simulink model "LKAS_DFL_20210630"  (R2018b)
settings: Solver=FixedStepDiscrete  StartTime=0.0  StopTime=10.0  FixedStep=0.01  RelTol=1e-3
InitFcn:
  | tmpVer = ver('MATLAB');
  | tmpVer = str2num(tmpVer.Version);
  | % -------------------------------------------------------------------
  | %  MATLAB file generated by Simulink.saveVars on 21-Nov-2019 10:06:14
  | %  MATLAB version: 7.13.0.564 (R2011b)
  | % -------------------------------------------------------------------
  | 
  | 
  | SInt16 = Simulink.AliasType;
  | SInt16.Description = 'Num';
  | if (tmpVer > 7.11)
  | 	SInt16.DataScope = 'Auto';
  | end
  | SInt16.HeaderFile = 'Rte_Type.h';
  | SInt16.BaseType = 'int16';
  | 
  | SInt32 = Simulink.AliasType;
  | SInt32.Description = 'Num';
  | if (tmpVer > 7.11)
  | 	SInt32.DataScope = 'Auto';
  | end
  | SInt32.HeaderFile = 'Rte_Type.h';
  | SInt32.BaseType = 'int32';
  | 
  | SInt8 = Simulink.AliasType;
  | SInt8.Description = 'Num';
  | if (tmpVer > 7.11)
  | 	SInt8.DataScope = 'Auto';
  | end
  | SInt8.HeaderFile = 'Rte_Type.h';
  | SInt8.BaseType = 'int8';
  | 
  | T_A_m2_1024_1_u32 = Simulink.NumericType;
  | T_A_m2_1024_1_u32.Description = 'm2 (square meters  (m2))';
  | if (tmpVer > 7.11)
  | 	T_A_m2_1024_1_u32.DataScope = 'Auto';
  | end
  | T_A_m2_1024_1_u32.HeaderFile = 'Rte_Type.h';
  | T_A_m2_1024_1_u32.DataTypeMode = 'Fixed-point: slope and bias scaling';
  | T_A_m2_1024_1_u32.SignednessBool = false;
  | T_A_m2_1024_1_u32.WordLength = 32;
  | T_A_m2_1024_1_u32.FixedExponent = -10;
  | T_A_m2_1024_1_u32.SlopeAdjustmentFactor = 1;
  | T_A_m2_1024_1_u32.Bias = 0;
  | T_A_m2_1024_1_u32.DataTypeOverride = 'Inherit';
  | T_A_m2_1024_1_u32.IsAlias = true;
  | 
  | T_A_m2_65536_1_u16 = Simulink.NumericType;
  | T_A_m2_65536_1_u16.Description = 'm2 (square meters  (m2))';
  | if (tmpVer > 7.11)
  | 	T_A_m2_65536_1_u16.DataScope = 'Auto';
  | end
  | T_A_m2_65536_1_u16.HeaderFile = 'Rte_Type.h';
  | T_A_m2_65536_1_u16.DataTypeMode = 'Fixed-point: slope and bias scaling';
  | T_A_m2_65536_1_u16.SignednessBool = false;
  | T_A_m2_65536_1_u16.WordLength = 16;
  | T_A_m2_65536_1_u16.FixedExponent = -16;
  | T_A_m2_65536_1_u16.SlopeAdjustmentFactor = 1;
  | T_A_m2_65536_1_u16.Bias = 0;
  | T_A_m2_65536_1_u16.DataTypeOverride = 'Inherit';
  | ... (+4598 lines)
StopFcn:
  | clear  T_A_m2_1024_1_u32 T_A_m2_65536_1_u16 T_A_m2_Float32 T_A_mm2_10_1_u16 T_A_mm2_4_1_s16 T_A_mm2_Float32 T_Cnt_Num_10_1_u32 T_Cnt_Num_1_1_s16 T_Cnt_Num_1_1_s32 T_Cnt_Num_1_1_s8 T_Cnt_Num_1_1_u16 T_Cnt_Num_1_1_u32 T_Cnt_Num_1_1_u8 T_E_J_1_1_s32 T_E_J_Float32 T_E_kJ_128_1_s32 T_E_kJ_Float32 T_E_kwh_10_1_u16 T_E_kwh_Float32 T_Epl_kwhpkm_100_1_u16 T_Epl_kwhpkm_Float32 T_F_N_1_1_s16 T_F_N_Float32 T_I_A_1000_1_u16 T_I_A_1048576_1_s32 T_I_A_2048_1_s16 T_I_A_32_1_s16 T_I_A_Float32 T_I_mA_1_1_s16 T_I_mA_32768_128_s16 T_I_mA_Float32 T_J_kgpm2_128_1_u16 T_J_kgpm2_Float32 T_K_NA_1000_1_s16 T_K_NA_100_1_s16 T_K_NA_100_1_u16 T_K_NA_1024_1_s16 T_K_NA_1024_1_u16 T_K_NA_128_1_s16 T_K_NA_128_1_u16 T_K_NA_128_1_u8 T_K_NA_16777216_1_u32 T_K_NA_16_1_s16 T_K_NA_16_1_u16 T_K_NA_16_1_u8 T_K_NA_1_16_u16 T_K_NA_1_1_s16 T_K_NA_1_1_u16 T_K_NA_1_1_u8 T_K_NA_32768_1_s16 T_K_NA_32768_1_u16 T_K_NA_32_1_s8 T_K_NA_4096_1_u16 T_K_NA_4194304_1_s32 T_K_NA_4194304_1_u16 T_K_NA_65536_1_s32 T_K_NA_65536_1_u16 T_K_NA_8192_1_s16 T_K_NA_8_1_s16 T_K_NA_Float32 T_M_Nm_16_1_s16 T_M_Nm_1_1_s16 T_M_Nm_32768_1_s16 T_M_Nm_32_1_s16 T_M_Nm_4_1_s16 T_M_Nm_512_1_s16 T_M_Nm_Float32 T_P_W_1_4_s16 T_P_W_1_8_s16 T_P_W_Float32 T_P_kW_128_1_s16 T_P_kW_1_8_s16 T_P_kW_8_1_s32 T_P_kW_Float32 T_Pct_pct_1024_1_s32 T_Pct_pct_1024_1_u32 T_Pct_pct_10_1_s16 T_Pct_pct_10_1_u32 T_Pct_pct_128_100_s8 T_Pct_pct_1_1_s16 T_Pct_pct_1_4_u8 T_Pct_pct_255_100_u16 T_Pct_pct_255_100_u8 T_Pct_pct_256_1_s16 T_Pct_pct_256_1_u16 T_Pct_pct_65535_100_u16 T_Pct_pct_Float32 T_R_ohm_1024_1_s16 T_R_ohm_32_1_s16 T_R_ohm_Float32 T_TK_K_16_1_s16 T_TK_K_Float32 T_T_degC_10_400_1_u16 T_T_degC_16_1_s16 T_T_degC_1_40_1_u8 T_T_degC_2_80_1_u8 T_T_degC_Float32 T_U_V_1000_1_u16 T_U_V_10_1_u8 T_U_V_200_1_u8 T_U_V_32_1_s16 T_U_V_4096_1_s16 T_U_V_512_1_s16 T_U_V_65535_8_u16 T_U_V_8192_1_u16 T_U_V_Float32 T_U_mV_1_1_s16 T_U_mV_256_20_u16 T_U_mV_Float32 T_V_l_256_1_s16 T_V_l_4096_1_s16 T_V_l_64_1_s16 T_V_l_65535_100_u16 T_V_l_Float32 T_V_ml_128_1_s16 T_V_ml_1_1_s16 T_V_ml_32768_1_s16 T_V_ml_Float32 T_V_ul_32_1_u16 T_V_ul_Float32 T_Vpl_clpkm_512_1_u16 T_Vpl_clpkm_Float32 T_a_kphps_16_1_s16 T_a_kphps_Float32 T_a_mps2_128_1_s16 T_a_mps2_Float32 T_c_MJpkg_256_1_s16 T_c_MJpkg_Float32 T_c_kJpgpK_1024_1_s16 T_c_kJpgpK_Float32 T_c_kJpkgpK_128_1_u16 T_c_kJpkgpK_Float32 T_chrg_Ah_1_1_s16 T_chrg_Ah_1_1_u16 T_chrg_Ah_1_1_u8 T_chrg_Ah_256_1_u16 T_chrg_Ah_4194304_1_s32 T_chrg_Ah_512_1_u16 T_chrg_Ah_8_1_u16 T_chrg_Ah_Float32 T_cmp_NA_100_1_s16 T_cmp_NA_128_1_s16 T_cmp_NA_16_1_s16 T_cmp_NA_32768_1_u16 T_cmp_NA_Float32 T_d2n_rpmps2_4_1_s16 T_d2n_rpmps2_Float32 T_dPct_pctps_16_1_s16 T_dPct_pctps_256_1_s16 T_dPct_pctps_Float32 T_dT_degCps_128_1_s16 T_dT_degCps_Float32 T_dV_lph_1_1_s16 T_dV_lph_Float32 T_dV_lpm_128_1_s16 T_dV_lpm_32_1_s16 T_dV_lpm_Float32 T_dV_lps_1024_1_u16 T_dV_lps_4_1_u16 T_dV_lps_Float32 T_dV_mlps_1024_1_s16 T_dV_mlps_Float32 T_d_BitField16 T_dm_gps_128_1_s16 T_dm_gps_128_1_u16 T_dm_gps_256_1_u16 T_dm_gps_Float32 T_dm_mgps_1_1_s16 T_dm_mgps_Float32 T_dn_rpmps_1_1_s16 T_dn_rpmps_2_1_s16 T_dn_rpmps_Float32 T_dp_Paps_1_1_s16 T_dp_Paps_Float32 T_dp_kPaps_1_1_s16 T_dp_kPaps_8_1_s16 T_dp_kPaps_Float32 T_dphi_degps_128_1_s16 T_dphi_degps_8_1_s16 T_dphi_degps_Float32 T_dr_ps_256_1_s16 T_dr_ps_Float32 T_drho_mgplps_1_2_s16 T_drho_mgplps_Float32 T_e_NA_1_1_u8 T_f_Hz_1_1_u16 T_f_Hz_1_1_u32 T_f_Hz_64_1_u16 T_f_Hz_8_1_s16 T_f_Hz_Float32 T_g_BitField32 T_l_km_16_1_s16 T_l_km_1_1_u16 T_l_km_1_1_u32 T_l_km_Float32 T_l_m_1024_1_s16 T_l_m_16_1_s16 T_l_m_1_1_u32 T_l_m_Float32 T_l_mm_16_1_s16 T_l_mm_1_1_u16 T_l_mm_4096_1_s16 T_l_mm_4_1_u8 T_l_mm_64_1_s16 T_l_mm_Float32 T_m_g_1_1_s16 T_m_g_2048_1_s16 T_m_g_32_1_u16 T_m_g_Float32 T_m_kg_1024_1_s16 T_m_kg_1_1_s16 T_m_kg_1_1_u32 T_m_kg_Float32 T_m_mg_128_1_s16 T_m_mg_32_1_s16 T_m_mg_Float32 T_n_rpm_1_1_s16 T_n_rpm_1_25_u8 T_n_rpm_256_50_u16 T_n_rpm_2_25_u8 T_n_rpm_4_1_u16 T_n_rpm_Float32 T_p_MPa_64_1_s16 T_p_MPa_Float32 T_p_Pa_1_1_s16 T_p_Pa_Float32 T_p_kPa_1_10_u16 T_p_kPa_1_1_s16 T_p_kPa_1_1_u8 T_p_kPa_256_1_u16 T_p_kPa_32_1_u16 T_p_kPa_64_1_s16 T_p_kPa_Float32 T_phi_deg_100_1_s16 T_phi_deg_1024_1_s16 T_phi_deg_128_1_s16 T_phi_deg_1_1_u8 T_phi_deg_256_1_s16 T_phi_deg_2_1_s8 T_phi_deg_32_1_s16 T_phi_deg_512_6_s32 T_phi_deg_Float32 T_phi_rad_2048_1_s16 T_phi_rad_Float32 T_r_NA_1024_1_s16 T_r_NA_1024_1_u16 T_r_NA_16384_1_s16 T_r_NA_16_1_s16 T_r_NA_256_1_s8 T_r_NA_256_1_u16 T_r_NA_32768_1_u16 T_r_NA_32_1_u16 T_r_NA_4096_1_s16 T_r_NA_65535_2_u16 T_r_NA_8192_1_u16 T_r_NA_Float32 T_rho_gpl_8192_1_s16 T_rho_gpl_Float32 T_rho_kgpm3_16_1_s16 T_rho_kgpm3_Float32 T_rho_mgpl_1_1_s16 T_rho_mgpl_64_1_s16 T_rho_mgpl_Float32 T_t_hour_1_1_s16 T_t_hour_Float32 T_t_m_1_1_u16 T_t_m_Float32 T_t_ms_1_1_s16 T_t_ms_1_1_u16 T_t_ms_1_1_u32 T_t_ms_4096_1_s16 T_t_ms_64_1_s16 T_t_ms_Float32 T_t_s_1000_1_s16 T_t_s_100_1_s16 T_t_s_10_1_s16 T_t_s_10_1_u16 T_t_s_1_1_s16 T_t_s_1_1_u16 T_t_s_1_1_u32 T_t_s_Float32 T_t_us_10_1_u32 T_t_us_1_1_s16 T_t_us_1_1_u32 T_t_us_1_4_u16 T_t_us_Float32 T_v_kph_1_1_u8 T_v_kph_64_1_s16 T_v_kph_64_1_u16 T_v_kph_Float32 T_v_mps_256_1_s16 T_v_mps_Float32 T_w_radps_32_1_s16 T_w_radps_Float32 T_y_BitField8 T_y_BitFieldDiagProgress T_y_BitFieldDiagStatus T_y_NA_1_1_u8 SInt16 SInt32 SInt8 T_BOOLEAN UInt16 UInt32 UInt8 s16 s32 s8 u16 u32 u8
model workspace (MAT data in the model file):
  MCOS : class17 (value not decoded)
  MCOS : class17 (value not decoded)
  MCOS : class17 (value not decoded)
  MCOS : class17 (value not decoded)
  MCOS : class17 (value not decoded)
  MCOS : class17 (value not decoded)
  MCOS : class17 (value not decoded)
  MCOS : class17 (value not decoded)
  MCOS : class17 (value not decoded)
  MCOS : class17 (value not decoded)
  MCOS : class17 (value not decoded)
  MCOS : class17 (value not decoded)
  MCOS : class17 (value not decoded)
  MCOS : class17 (value not decoded)
  MCOS : class17 (value not decoded)
  MCOS : class17 (value not decoded)
  MCOS : class17 (value not decoded)
  MCOS : class17 (value not decoded)
  MCOS : class17 (value not decoded)
  MCOS : class17 (value not decoded)
  MCOS : class17 (value not decoded)
  MCOS : class17 (value not decoded)
  MCOS : class17 (value not decoded)
  MCOS : class17 (value not decoded)
  MCOS : class17 (value not decoded)
  MCOS : class17 (value not decoded)
  MCOS : class17 (value not decoded)
  MCOS : class17 (value not decoded)
  MCOS : class17 (value not decoded)
  MCOS : class17 (value not decoded)
  MCOS : class17 (value not decoded)
  MCOS : class17 (value not decoded)
  MCOS : class17 (value not decoded)
  MCOS : class17 (value not decoded)
  MCOS : class17 (value not decoded)
  MCOS : class17 (value not decoded)
  MCOS : class17 (value not decoded)
  MCOS : class17 (value not decoded)
  MCOS : class17 (value not decoded)
  MCOS : class17 (value not decoded)
  MCOS : class17 (value not decoded)
  MCOS : class17 (value not decoded)
  MCOS : class17 (value not decoded)
  MCOS : class17 (value not decoded)
  MCOS : class17 (value not decoded)
  MCOS : class17 (value not decoded)
  MCOS : class17 (value not decoded)
  MCOS : class17 (value not decoded)
  MCOS : class17 (value not decoded)
  MCOS : class17 (value not decoded)
  MCOS : class17 (value not decoded)
  MCOS : class17 (value not decoded)
  MCOS : class17 (value not decoded)
  MCOS : class17 (value not decoded)
  MCOS : class17 (value not decoded)
  MCOS : class17 (value not decoded)
  MCOS : class17 (value not decoded)
  MCOS : class17 (value not decoded)
  MCOS : class17 (value not decoded)
  MCOS : class17 (value not decoded)
  MCOS : class17 (value not decoded)
  MCOS : class17 (value not decoded)
  MCOS : class17 (value not decoded)
  MCOS : class17 (value not decoded)
  MCOS : class17 (value not decoded)
  MCOS : class17 (value not decoded)
  MCOS : class17 (value not decoded)
  MCOS : class17 (value not decoded)
  MCOS : class17 (value not decoded)
  MCOS : class17 (value not decoded)
  MCOS : class17 (value not decoded)
  MCOS : class17 (value not decoded)
  MCOS : class17 (value not decoded)
  MCOS : class17 (value not decoded)
  MCOS : class17 (value not decoded)
  MCOS : class17 (value not decoded)
  MCOS : class17 (value not decoded)
  MCOS : class17 (value not decoded)
  MCOS : class17 (value not decoded)
  MCOS : class17 (value not decoded)
  MCOS : class17 (value not decoded)
  MCOS : class17 (value not decoded)
  MCOS : class17 (value not decoded)
  MCOS : class17 (value not decoded)
  MCOS : class17 (value not decoded)
  MCOS : class17 (value not decoded)
  MCOS : class17 (value not decoded)
  MCOS : class17 (value not decoded)
  MCOS : class17 (value not decoded)
  MCOS : class17 (value not decoded)
  MCOS : class17 (value not decoded)
  MCOS : class17 (value not decoded)
  MCOS : class17 (value not decoded)
  MCOS : class17 (value not decoded)
  MCOS : class17 (value not decoded)
undefined symbols (not defined in the file): LKA_CarWidth, LKA_SampleTime, LKA_StrRatio_C, LKA_Veh2CamL_C, LKA_Veh2CamW_C, LKA_WhlBaseL_C, LL_CompSWA_C, LL_CrvtPrvwT_C, LL_DesDvt_C, LL_DvtComp_C, LL_DvtPrvwT_C, LL_DvtSpdDet_vDvtSpdMin_C, LL_HdAgExT_C, LL_HdAgPrvwT_C, LL_LAccMax_C, LL_LAccRMax_C, LL_Laneline_Select, LL_LDW_EarliestWarnLine_C, LL_LDW_LatestWarnLine_C, LL_LDWS_SUPPRESS_HEADING, LL_LFClb_TFC_DiffCtlBalance, LL_LFClb_TFC_DiffCtrlMaxSWA, LL_LFClb_TFC_DiffCtrlRatio, LL_LFClb_TFC_facmGainLutGain1_C, LL_LFClb_TFC_facmGainLutGain2_C, LL_LFClb_TFC_facmIntegRatio, LL_LFClb_TFC_facmKlat_C, LL_LFClb_TFC_FfCtlRatio_C, LL_LFClb_TFC_phiIntegCtlMaxSWA_C, LL_LFClb_TFC_tiKlatPrvwT_C, LL_LFClb_TFC_vGainLutVehSpdLwr_C, LL_LFClb_TFC_vGainLutVehSpdUpr_C, LL_LKA_EarliestWarnLine_C, LL_LKA_LatestWarnLine_C, LL_LKAExPrcs_ExitC0Dvt, LL_LKAExPrcs_ExitC0Swt, LL_LKAExPrcs_tiExitTime1, LL_LKAExPrcs_tiExitTime2, LL_LKAExPrcs_tiExitTime3, LL_LKAS_OUT_OF_CONTROL_LAT_VEL, LL_LKAS_OUT_OF_CONTROL_TTLC, LL_LKASWASyn_M0, LL_LKASWASyn_M1, LL_LKASWASyn_M2, LL_LKASWASyn_M3K, LL_LKASWASyn_SWAaddMax, LL_LKASWASyn_T2, LL_LKASWASyn_tiTrqSwaRtTime, LL_LKASWASyn_tiTrqSwaTime, LL_LKASWASyn_TrqMax, LL_LKASWASyn_TrqSwaAddSwt, LL_LKASWASyn_TrqSwaRateDiff, LL_LSpdCompT_C, LL_lStpLngth_C, LL_MAX_DELAY_EPSSTAR_TIME, LL_MAX_DRIVER_TORQUE_DISABLE, LL_MAX_DRIVER_TORQUE_ENABLE, LL_MAX_LANE_WIDTH_DISABLE, LL_MAX_LANE_WIDTH_ENABLE, LL_MAX_LAT_ACC_DISABLE ... (+35)
libraries: simulink x130, dspstat3 x3, simulink_extras x1
(part 6 of 18)

== system LKAS_DFL_20210630/LKAS/LL/LL Inputs Mapping/bsBCMInfo ==
  note: <BCM_Double_Light>
      | 0:off
      | 1:on
  note: <BCM_Left_Light>
      | 0:off
      | 1:on
  note: <BCM_Right_Light>
      | 0:off
      | 1:on
  bsBCMInfoIn : Inport
  Bus Creator1 : BusCreator  Inputs=3
  Bus Selector1 : BusSelector  OutputSignals=BCM_Double_Light,BCM_Left_Light,BCM_Right_Light
  bsBCMInfoOut : Outport
  wires:
  Bus Selector1/3 -> Bus Creator1/3  "<BCM_Right_Light>"
  Bus Selector1/2 -> Bus Creator1/2  "<BCM_Left_Light>"
  Bus Creator1/1 -> bsBCMInfoOut/1
  Bus Selector1/1 -> Bus Creator1/1  "<BCM_Double_Light>"
  bsBCMInfoIn/1 -> Bus Selector1/1

== system LKAS_DFL_20210630/LKAS/LL/LL Inputs Mapping/bsEPSInfo ==
  note: <EPS_LKA_State>
      | 0:init
      | 1:authorized
      | 2:wait
      | 3:active
      | 4:fault
  note: <EPS_Error_State>
      | 0:no error
      | 1:error
  note: <EPS_Trq_State>
      | 0:no error
      | 1:error
  note: <SAS_Clb_State>
      | 0:no clb
      | 1:clb
  note: <SAS_Trim_State>
      | 0:no trim
      | 1:trim
  note: <EPS_TrqLim_State>
      | 0:no limit
      | 1:limit
  note: <EPS_SWHold_State>
      | 0:no hold
      | 1:hold
  bsEPSInfoIn : Inport
  Bus Creator4 : BusCreator  Inputs=9
  Bus Selector1 : BusSelector  OutputSignals=EPS_LKA_State,EPS_SW_Trq,EPS_Error_State,EPS_Trq_State,SAS_Clb_State,SAS_Trim_State,EPS_TrqLim_State,EPS_LKA_Current,EPS_SWHold_State
  bsEPSInfoOut : Outport
  wires:
  Bus Selector1/9 -> Bus Creator4/9  "<EPS_SWHold_State>"
  Bus Selector1/8 -> Bus Creator4/8  "<EPS_LKA_Current>"
  Bus Selector1/7 -> Bus Creator4/7  "<EPS_TrqLim_State>"
  Bus Selector1/6 -> Bus Creator4/6  "<SAS_Trim_State>"
  Bus Selector1/5 -> Bus Creator4/5  "<SAS_Clb_State>"
  Bus Selector1/4 -> Bus Creator4/4  "<EPS_Trq_State>"
  Bus Selector1/3 -> Bus Creator4/3  "<EPS_Error_State>"
  Bus Creator4/1 -> bsEPSInfoOut/1
  Bus Selector1/1 -> Bus Creator4/1  "<EPS_LKA_State>"
  Bus Selector1/2 -> Bus Creator4/2  "<EPS_SW_Trq>"
  bsEPSInfoIn/1 -> Bus Selector1/1

== system LKAS_DFL_20210630/LKAS/LL/LL Inputs Mapping/bsLaneInfo ==
  bsLaneInfoIn : Inport
  Bus Creator : BusCreator  Inputs=7
  Bus Selector1 : BusSelector  OutputSignals=bsFusLaneInfo,bsFusL0Info,bsFusR0Info,bsFusL1Info,bsFusR1Info,bsOriLaneInfo,bsOriL0Info,bsOriR0Info,bsOriL1Info,bsOriR1Info,Fusion_AdditionalInf
  LaneSelect : Subsystem
  "LanesReconstruct " : Subsystem
  bsLaneInfoOut : Outport
  wires:
  Bus Selector1/1 -> Bus Creator/1  "<bsFusLaneInfo>"
  Bus Selector1/6 -> Bus Creator/6  "<bsOriLaneInfo>"
  Bus Creator/1 -> bsLaneInfoOut/1
  Bus Selector1/10 -> LaneSelect/8(bsOriR1Info)  "<bsOriR1Info>"
  Bus Selector1/9 -> LaneSelect/7(bsOriL1Info)  "<bsOriL1Info>"
  Bus Selector1/8 -> LaneSelect/6(bsOriR0Info)  "<bsOriR0Info>"
  Bus Selector1/7 -> LaneSelect/5(bsOriL0Info)  "<bsOriL0Info>"
  Bus Selector1/5 -> LaneSelect/4(bsFusR1Info)  "<bsFusR1Info>"
  Bus Selector1/4 -> LaneSelect/3(bsFusL1Info)  "<bsFusL1Info>"
  Bus Selector1/3 -> LaneSelect/2(bsFusR0Info)  "<bsFusR0Info>"
  Bus Selector1/2 -> LaneSelect/1(bsFusL0Info)  "<bsFusL0Info>"
  LaneSelect/4(bsR1Info) -> "LanesReconstruct "/4(bsR1Info)
  LaneSelect/3(bsL1Info) -> "LanesReconstruct "/3(bsL1Info)
  LaneSelect/2(bsR0Info) -> "LanesReconstruct "/2(bsR0Info)
  LaneSelect/1(bsL0Info) -> "LanesReconstruct "/1(bsL0Info)
  "LanesReconstruct "/4(bsR1InfoR) -> Bus Creator/5  "bsR1Info"
  "LanesReconstruct "/3(bsL1InfoR) -> Bus Creator/4  "bsL1Info"
  "LanesReconstruct "/2(bsR0InfoR) -> Bus Creator/3  "bsR0Info"
  "LanesReconstruct "/1(bsL0InfoR) -> Bus Creator/2  "bsL0Info"
  Bus Selector1/11 -> Bus Creator/7  "<Fusion_AdditionalInf>"
  bsLaneInfoIn/1 -> Bus Selector1/1

== system LKAS_DFL_20210630/LKAS/LL/LL Inputs Mapping/bsMP5Info ==
  note: <LKA_Main_Switch>
      | 0:off
      | 1:on
  note: <LKA_Mode>
      | 0:off
      | 1:LDW
      | 2:LKA
  bsMP5InfoIn : Inport
  Add : Sum
  Bus Selector1 : BusSelector  OutputSignals=LKA_Main_Switch,LKA_Mode
  Constant : Constant  OutDataTypeStr=uint8
  Divide : Product  Inputs=**  OutDataTypeStr=uint8
  stDACMode : Outport
  wires:
  bsMP5InfoIn/1 -> Bus Selector1/1
  Divide/1 -> stDACMode/1
  Bus Selector1/1 -> Divide/1  "<LKA_Main_Switch>"
  Bus Selector1/2 -> Add/1  "<LKA_Mode>"
  Constant/1 -> Add/2
  Add/1 -> Divide/2  "LKA_Mode"

== system LKAS_DFL_20210630/LKAS/LL/LL Inputs Mapping/bsPTState ==
  note: <TCU_ActualGear>
      | 0： P
      | 1： R
      | 2： N
      | 3： D
  bsPTStateIn : Inport
  Bus Creator3 : BusCreator  Inputs=2
  Bus Selector1 : BusSelector  OutputSignals=AccPedal_Pos,TCU_ActualGear
  MATLAB Function : MATLAB Function  TreatAsAtomicUnit=on
  bsPTStateOut : Outport
  wires:
  Bus Creator3/1 -> bsPTStateOut/1
  Bus Selector1/1 -> Bus Creator3/1  "<AccPedal_Pos>"
  bsPTStateIn/1 -> Bus Selector1/1
  Bus Selector1/2 -> MATLAB Function/1(u)  "<TCU_ActualGear>"
  MATLAB Function/1(y) -> Bus Creator3/2  "TCU_ActualGear"

== system LKAS_DFL_20210630/LKAS/LL/LL Inputs Mapping/bsSWAInfo ==
  note: <SWS_Fault_Code>
      | 0:no error
      | 1:error1
      | 2:error2
  note: <SWS_Failure_Status>
      | 0:no error
      | 1:error
  bsSWAInfoIn : Inport
  Bus Creator : BusCreator  Inputs=4
  Bus Selector1 : BusSelector  OutputSignals=SW_Angle,SW_Angle_Speed,SWS_Fault_Code,SWS_Failure_Status
  bsSWAInfoOut : Outport
  wires:
  Bus Creator/1 -> bsSWAInfoOut/1
  Bus Selector1/4 -> Bus Creator/4  "<SWS_Failure_Status>"
  Bus Selector1/3 -> Bus Creator/3  "<SWS_Fault_Code>"
  Bus Selector1/2 -> Bus Creator/2  "<SW_Angle_Speed>"
  Bus Selector1/1 -> Bus Creator/1  "<SW_Angle>"
  bsSWAInfoIn/1 -> Bus Selector1/1

== system LKAS_DFL_20210630/LKAS/LL/LL Inputs Mapping/bsVehMovInfo ==
  note: <ESC_LatAcc_Valid>
      | 0:invalid
      | 1:valid
  note: <ESC_YawRate_Valid>
      | 0:invalid
      | 1:valid
  note: <ESC_LonAcc_Valid>
      | 0:invalid
      | 1:valid
  note: <ESC_VehSpd_Valid>
      | 0:invalid
      | 1:valid
  bsVehMovInfoIn : Inport
  Bus Creator : BusCreator  Inputs=10
  Bus Selector2 : BusSelector  OutputSignals=ESC_LatAcc,ESC_LatAcc_Valid,ESC_YawRate,ESC_YawRate_Valid,ESC_UnYawRate,ESC_VehSpd,ESC_LonAcc,ESC_LonAcc_Valid,ESC_Brake_Press,ESC_VehSpd_Valid
  bsVehMovInfoOut : Outport
  wires:
  Bus Creator/1 -> bsVehMovInfoOut/1
  Bus Selector2/10 -> Bus Creator/10  "<ESC_VehSpd_Valid>"
  Bus Selector2/9 -> Bus Creator/9  "<ESC_Brake_Press>"
  Bus Selector2/8 -> Bus Creator/8  "<ESC_LonAcc_Valid>"
  Bus Selector2/7 -> Bus Creator/7  "<ESC_LonAcc>"
  Bus Selector2/6 -> Bus Creator/6  "<ESC_VehSpd>"
  Bus Selector2/5 -> Bus Creator/5  "<ESC_UnYawRate>"
  Bus Selector2/4 -> Bus Creator/4  "<ESC_YawRate_Valid>"
  Bus Selector2/3 -> Bus Creator/3  "<ESC_YawRate>"
  Bus Selector2/2 -> Bus Creator/2  "<ESC_LatAcc_Valid>"
  Bus Selector2/1 -> Bus Creator/1  "<ESC_LatAcc>"
  bsVehMovInfoIn/1 -> Bus Selector2/1

== system LKAS_DFL_20210630/LKAS/LL/LLOn/LDW ==
  LDW_bsInInfoSyn : Inport
  LDW_bsLDWClb : Inport  Port=2
  Enable : EnablePort  StatesWhenEnabling=reset  ShowOutputPort=on
      settings: AttributesFormatString=states = %<StatesWhenEnabling>
  Bus Selector : BusSelector  OutputSignals=bsLaneInfo.bsL0Info.L0_C1,bsLaneInfo.bsR0Info.R0_C1
  Bus Selector1 : BusSelector  OutputSignals=bsLDWClb.LL_LDWS_SUPPRESS_HEADING,bsConstantClb.LKA_SampleTime
  Cast : DataTypeConversion  OutDataTypeStr=uint8
  Heading Angle Detection (HdAgDet) : Subsystem  Description=|
      | Block Name: Heading Angle Detection
      | Ab.: HdAgDet
      | No.: 1.3.1.0
      | Rev: 0.0.1
      | Update Date: 19-3-26
  Logical Operator : Logic  Operator=NOT  AllPortsSameDT=off  OutDataTypeStr=boolean
  Product : Product  OutDataTypeStr=uint8
  LDW_Flag : Outport  OutputWhenDisabled=reset  InitialOutput=0
      settings: AttributesFormatString=%<OutputWhenDisabled> = %<InitialOutput>
  wires:
  Logical Operator/1 -> Cast/1
  Cast/1 -> Product/2
  Bus Selector1/2 -> Heading Angle Detection (HdAgDet)/5(SampleTime)  "<LKA_SampleTime>"
  Product/1 -> LDW_Flag/1
  Heading Angle Detection (HdAgDet)/1(HdAgDet_stHdAgDetFlg) -> Logical Operator/1
  LDW_bsInInfoSyn/1 -> Bus Selector/1
  Enable/1 -> Heading Angle Detection (HdAgDet)/1(HdAgDet_stLDWActvFlg), Product/1
  Bus Selector/1 -> Heading Angle Detection (HdAgDet)/2(HdAgDet_phiHdAgLft)  "<L0_C1>"
  Bus Selector/2 -> Heading Angle Detection (HdAgDet)/3(HdAgDet_phiHdAgRgt)  "<R0_C1>"
  LDW_bsLDWClb/1 -> Bus Selector1/1
  Bus Selector1/1 -> Heading Angle Detection (HdAgDet)/4(HdAgDet_phiHdAgThres_C)  "<LL_LDWS_SUPPRESS_HEADING>"

== system LKAS_DFL_20210630/LKAS/LL/LLOn/LKA ==
  LKA_bsInInfoSyn : Inport
  LKA_bsLKAInPInfo : Inport  Port=2
  LKA_bsLKAClb : Inport  Port=3
  Enable : EnablePort  StatesWhenEnabling=reset  ShowOutputPort=on
      settings: AttributesFormatString=states = %<StatesWhenEnabling>
  Bus Selector : BusSelector  OutputSignals=bsConstantClb.LKA_SampleTime
  Cast To Single : DataTypeConversion  OutDataTypeStr=uint8
  Driver Torque Addition (DTA) : Subsystem
  LKA Exit Processing (LKAExPrcs) : Subsystem  Description=|
      | Block Name: LKA Exit Processing 
      | Ab.: LKAExPrcs
      | No.: 1.2.2.0
      | Rev: 0.0.1
      | Update Date: 19-5-13
  "LKA Motion Planning (LKAMP) " : Subsystem  Description=|
      | Block Name: LKA Motion Planning
      | Ab.: LKAMP
      | No.: 1.2.3.0
      | Rev: 0.0.1
      | Update Date: 19-5-13
  LKA SWA Limit (LKASWALim) : Subsystem  Description=|
      | Block Name: LKA SWA Synthesis
      | Ab.: LKASWASyn
      | No.: 1.2.6.0
      | Rev: 0.0.1
      | Update Date: 19-5-13
  LKA_Mon : Subsystem
  Lane Following (LF) : Subsystem  Description=|
      | Block Name: Lane Following
      | Ab.: LF
      | No.: 02
      | Rev: 00.00.01
      | Update Date: 19-3-28
  Plan To LaneFollowing (PTLF) : Subsystem
  LKA_ExitFlg : Outport  OutputWhenDisabled=reset  InitialOutput=0
      settings: AttributesFormatString=%<OutputWhenDisabled> = %<InitialOutput>
  LKA_phiSWACmd : Outport  Port=2  OutputWhenDisabled=reset  InitialOutput=0
      settings: AttributesFormatString=%<OutputWhenDisabled> = %<InitialOutput>
  LKA_M : Outport  Port=3  OutputWhenDisabled=reset  InitialOutput=0
      settings: AttributesFormatString=%<OutputWhenDisabled> = %<InitialOutput>
  LKAMon : Outport  Port=4  OutputWhenDisabled=reset  InitialOutput=0
      settings: AttributesFormatString=%<OutputWhenDisabled> = %<InitialOutput>
  tag scope: ActFlg=global, Ff=global, LKA_ExitFlg_Mon=global, LKA_SampleTime=global, PT1=global
  wires:
  Cast To Single/1 -> [ActFlg]  "ActFlg"
  Plan To LaneFollowing (PTLF)/1(SWACmd) -> LKA SWA Limit (LKASWALim)/1(LKASWALim_phiTFCSWACmd)  "PTLFSWACmd"
  Enable/1 -> Cast To Single/1
  LKA SWA Limit (LKASWALim)/1(LKASWALim_phiSWACmd) -> LKA_phiSWACmd/1  "phiSWACmd"
  LKA Exit Processing (LKAExPrcs)/1(LKAExPrcs_stExFlg) -> LKA_ExitFlg/1, [LKA_ExitFlg_Mon]
  [Ff] -> Plan To LaneFollowing (PTLF)/5(Ff)
  [P] -> Plan To LaneFollowing (PTLF)/6(P)
  [I] -> Plan To LaneFollowing (PTLF)/7(I)
  [D] -> Plan To LaneFollowing (PTLF)/8(D)
  Driver Torque Addition (DTA)/1(DTA_phiDTASWACmd) -> [DT]  "DT"
  [DT] -> Plan To LaneFollowing (PTLF)/4(DrvTrq)
  [Plan] -> Plan To LaneFollowing (PTLF)/2(Plan)
  [PT1] -> Plan To LaneFollowing (PTLF)/3(T1)
  [PT1] -> LKA Exit Processing (LKAExPrcs)/3(LKAExPrcs_PlanT1)
  [ActFlg] -> "LKA Motion Planning (LKAMP) "/2(LKAMP_stLKAActvFlg)
  LKA_bsLKAInPInfo/1 -> [LKAInPInfo]
  [LKAInPInfo] -> "LKA Motion Planning (LKAMP) "/3(LKAMP_bsLKAInPInfo)
  [LKAInPInfo] -> LKA Exit Processing (LKAExPrcs)/1(LKAExPrcs_bsLKAInPInfo)
  [LKAInPInfo] -> Plan To LaneFollowing (PTLF)/1(InP)
  LKA_bsLKAClb/1 -> Bus Selector/1, [LKA_bsLLClb]
  [LKAInPInfo] -> LKA SWA Limit (LKASWALim)/3(LKASWALim_bsLKAInPInfo)
  [LKA_bsLLClb] -> LKA Exit Processing (LKAExPrcs)/2(LKAExPrcs_bsLKAClb)
  [LKA_bsLLClb] -> Driver Torque Addition (DTA)/2(DTA_bsLFClb)
  [LKA_bsLLClb] -> Lane Following (LF)/3(LF_bsLFClb)
  [LKA_bsLLClb] -> LKA SWA Limit (LKASWALim)/4(LKASWALim_bsLKAClb)
  LKA_bsInInfoSyn/1 -> [LKA_bsInInfoSyn]
  [LKA_bsInInfoSyn] -> "LKA Motion Planning (LKAMP) "/1(LKAMP_bsInInfoSyn)
  [LKA_bsInInfoSyn] -> Driver Torque Addition (DTA)/1(DTA_bsInInfoSyn)
  [LKA_bsInInfoSyn] -> Lane Following (LF)/1(LF_bsInInfoSyn)
  [Ff] -> LKA SWA Limit (LKASWALim)/2(LKASWALim_Ff)
  [LKAInPInfo] -> Lane Following (LF)/2(LF_bsLKAInPInfo)
  Driver Torque Addition (DTA)/2(DTA_M) -> LKA_M/1
  Lane Following (LF)/3(LF_phiIntegSWACmd) -> [I]
  Lane Following (LF)/1(LF_phiFfLFSWACmd) -> [Ff]
  Lane Following (LF)/2(LF_phiPropSWACmd) -> [P]
  Lane Following (LF)/4(LF_phiDiffSWACmd) -> [D]
  "LKA Motion Planning (LKAMP) "/1(LKAMP_phiSWACmd) -> [Plan]  "PlanSWACmd"
  "LKA Motion Planning (LKAMP) "/3(LKAMP_tiT2) -> ?  "PlanT2"
  "LKA Motion Planning (LKAMP) "/2(LKAMP_tiT1) -> [PT1]  "PlanT1"
  LKA_Mon/1(LKAMon) -> LKAMon/1
  [LKA_bsLLClb] -> "LKA Motion Planning (LKAMP) "/4(LKAMP_bsLLClb)
  Bus Selector/1 -> [LKA_SampleTime]  "<LKA_SampleTime>"

== system LKAS_DFL_20210630/LKAS/LL/LLOn/LKA Input Processing (LKAInP) ==
  LKAInP_bsInInfoSyn : Inport
  LKAInP_bsLLClb : Inport  Port=2
  In3 : Inport  Port=3
  Bus Creator2 : BusCreator  Inputs=10
  Curvature Calculation (Crvt) : Subsystem
  Delay : Delay  DelayLength=1
  Deviation Calculation (Dvt) : Subsystem
  Heading Angle Calculation (HdAg) : Subsystem
  Lane Width Calculation (LW) : Subsystem
  Previewed Curvature Calculation (PrCrvt) : Subsystem
  Previewed Deviation Calculation (PrDvt) : Subsystem
  Previewed Heading Angle Calculation (PrHdAg) : Subsystem
  Steering Wheel Position Calculation (SWAPosCal) : Subsystem
  TTLC Calculation (TTLCCalc) : Subsystem  Description=|
      | Block Name: TTLC Calculation
      | Ab.: TTLCCalc
      | No.: 1.1.1.1
      | Rev: 0.0.1
      | Update Date: 19-3-26
  Under The Limit (UndrLim) : Subsystem
  LKAInP_bsLKAInPInfo : Outport
  wires:
  LKAInP_bsInInfoSyn/1 -> TTLC Calculation (TTLCCalc)/3(bsInfo), Previewed Deviation Calculation (PrDvt)/2(PrvwDvt_bsInInfoSyn), Previewed Heading Angle Calculation (PrHdAg)/1(PrHdAg_bsInInfoSyn), Previewed Curvature Calculation (PrCrvt)/1(PrvwCrvt_bsInInfoSyn), Deviation Calculation (Dvt)/1(Dvt_bsInInfoSyn), Heading Angle Calculation (HdAg)/1(HdAg_bsInInfoSyn), Under The Limit (UndrLim)/1(UndrLim_bsInInfoSyn), Steering Wheel Position Calculation (SWAPosCal)/1(SWAPosCal_bsInInfoSyn), Lane Width Calculation (LW)/1(LW_bsInInfoSyn), Curvature Calculation (Crvt)/1(PrvwCrvt_bsInInfoSyn)
  Heading Angle Calculation (HdAg)/1(HdAg_bsHdAgInfo) -> Bus Creator2/5  "bsHdAgInfo"
  LKAInP_bsLLClb/1 -> Previewed Heading Angle Calculation (PrHdAg)/2(PrHdAg_bsLLClb), Under The Limit (UndrLim)/2(UndrLim_bsLLClb), Steering Wheel Position Calculation (SWAPosCal)/2(SWAPosCal_bsLLClb), Deviation Calculation (Dvt)/2(Dvt_bsLLClb), Previewed Curvature Calculation (PrCrvt)/2(PrvwCrvt_tiCrvtPrvwT_C), TTLC Calculation (TTLCCalc)/2(bsLLClb), Previewed Deviation Calculation (PrDvt)/1(PrdcDvt_bsLLClb)
  Previewed Heading Angle Calculation (PrHdAg)/1(PrHdAg_bsPrHdAgInfo) -> Bus Creator2/8  "bsPrHdAgInfo"
  TTLC Calculation (TTLCCalc)/1(TTLCCalc_bsTTLCInfo) -> Previewed Heading Angle Calculation (PrHdAg)/3(PrHdAg_bsTTLCInfo), Bus Creator2/10  "bsTTLCInfo"
  Lane Width Calculation (LW)/1(LW_LaneWidth) -> Bus Creator2/1  "LaneWidth"
  Steering Wheel Position Calculation (SWAPosCal)/1(SWAPosCal) -> Bus Creator2/2  "phiSWAPos"
  Under The Limit (UndrLim)/1(UndrLim_bsUndrLimInfo) -> Bus Creator2/3  "bsUndrLimInfo"
  Deviation Calculation (Dvt)/1(Dvt_bsDvtInfo) -> TTLC Calculation (TTLCCalc)/1(bsDvtInfo), Bus Creator2/6  "bsDvtInfo"
  Curvature Calculation (Crvt)/1(Crvt_bsCrvtInfo) -> Bus Creator2/4  "bsCrvtInfo"
  Previewed Deviation Calculation (PrDvt)/1(PrvwDvt_bsPrvwDvtInfo) -> Bus Creator2/9  "bsPrDvtInfo"
  Previewed Curvature Calculation (PrCrvt)/1(PrvwCrvt_bsPrvwCrvtInfo) -> Bus Creator2/7, TTLC Calculation (TTLCCalc)/4(In4)  "bsPrCrvtInfo"
  Bus Creator2/1 -> LKAInP_bsLKAInPInfo/1
  In3/1 -> Delay/1
  Delay/1 -> Previewed Curvature Calculation (PrCrvt)/3(PrvwCrvt_stLKAActvFlg)

== system LKAS_DFL_20210630/LKAS/LL/LLOn/LL State Determination (LLStateDet) ==
  LLStateDet_bsInInfoSyn : Inport
  LLStateDet_bsLKAInPInfo : Inport  Port=2
  LLStateDet_bsLLClb : Inport  Port=3
  LLStateDet_stExitFlg : Inport  Port=4
  LLStateDet_SignalFault : Inport  Port=5
  Bus Creator : BusCreator  Inputs=3
  Delay : Delay  DelayLength=1
  Delay1 : Delay  DelayLength=1
  LDW_State_Machine : Stateflow chart  Description=|  TreatAsAtomicUnit=on
      | Block Name: LDW State Machine
      | Ab.: LDWSM
      | No.: 1.1.2.0
      | Rev: 0.0.1
      | Update Date: 19-3-26
      settings: RTWSystemCode=Nonreusable function
  LKA_State_Machine : Stateflow chart  Description=|  TreatAsAtomicUnit=on
      | Block Name: LKA State Machine
      | Ab.: LKASM
      | No.: 1.1.3.0
      | Rev: 0.0.1
      | Update Date: 19-3-26
      settings: RTWSystemCode=Nonreusable function
  LL State Machine Conditions (LLSMCon) : Subsystem
  LLStateDet_bsLLState : Outport
  LLStateDet_stLDWActvFlg : Outport  Port=2
  LLStateDet_stLKAActvFlg : Outport  Port=3
  Disable_Reason : Outport  Port=4
  tag scope: LDW_State_Mon=global, LKA_State_Mon=global
  wires:
  LL State Machine Conditions (LLSMCon)/2(LLSMCon_stLDWEnaCSyn) -> LDW_State_Machine/2(LDWSM_stEnaCSyn)
  LL State Machine Conditions (LLSMCon)/3(LLSMCon_stLDWDisblCSyn) -> LDW_State_Machine/3(LDWSM_stDisblCSyn)
  LL State Machine Conditions (LLSMCon)/4(LLSMCon_stLDWActvCSyn) -> LDW_State_Machine/4(LDWSM_stActvCSyn)
  LL State Machine Conditions (LLSMCon)/5(LLSMCon_stLDWDeactvCSyn) -> LDW_State_Machine/5(LDWSM_stDeactvCSyn)
  LL State Machine Conditions (LLSMCon)/1(LLSMCon_stDACMode) -> Bus Creator/2, LKA_State_Machine/1(LKASM_stLMCMode), LDW_State_Machine/1(LDWSM_stLMCMode)  "DACMode"
  LDW_State_Machine/1(LDWSM_stLDWActvFlg) -> LLStateDet_stLDWActvFlg/1
  LKA_State_Machine/1(LKASM_stLKAActvFlg) -> LLStateDet_stLKAActvFlg/1
  Delay1/1 -> LL State Machine Conditions (LLSMCon)/4(LLSMCon_bsLLState)
  Bus Creator/1 -> LLStateDet_bsLLState/1, Delay1/1  "LLState"
  LKA_State_Machine/2(LKASM_stLKAState) -> [LKA_State_Mon], Bus Creator/3  "LKA_State"
  LDW_State_Machine/2(LDWSM_stLDWState) -> [LDW_State_Mon], Bus Creator/1  "LDW_State"
  LL State Machine Conditions (LLSMCon)/6(LLSMCon_stLDWFaultCSyn) -> LDW_State_Machine/6(LDWSM_stFaultCSyn)
  LL State Machine Conditions (LLSMCon)/7(LLSMCon_stLKAEnaCSyn) -> LKA_State_Machine/2(LKASM_stEnaCSyn)
  LL State Machine Conditions (LLSMCon)/8(LLSMCon_stLKADisblCSyn) -> LKA_State_Machine/3(LKASM_stDisblCSyn)
  LL State Machine Conditions (LLSMCon)/9(LLSMCon_stLKAActvCSyn) -> LKA_State_Machine/4(LKASM_stActvCSyn)
  LL State Machine Conditions (LLSMCon)/10(LLSMCon_stLKADeactvCSyn) -> LKA_State_Machine/5(LKASM_stDeactvCSyn)
  LL State Machine Conditions (LLSMCon)/11(LLSMCon_stLKAFaultCSyn) -> LKA_State_Machine/6(LKASM_stFaultCSyn)
  LLStateDet_bsInInfoSyn/1 -> LL State Machine Conditions (LLSMCon)/1(LLSMCon_bsInInfoSyn)
  LLStateDet_bsLKAInPInfo/1 -> LL State Machine Conditions (LLSMCon)/2(LLSMCon_bsLKAInPInfo)
  LLStateDet_stExitFlg/1 -> Delay/1
  LLStateDet_bsLLClb/1 -> LL State Machine Conditions (LLSMCon)/3(LLSMCon_bsLLClb)
  Delay/1 -> LL State Machine Conditions (LLSMCon)/5(LLSMCon_stExitFlg)
  LLStateDet_SignalFault/1 -> LL State Machine Conditions (LLSMCon)/6(LLSMCon_bsSignalFault)
  LL State Machine Conditions (LLSMCon)/12(Disable_Reason) -> Disable_Reason/1

== system LKAS_DFL_20210630/LKAS/LL/LLOn/LL_Mon ==
  LKAMon : Inport
  Bus : BusCreator  Inputs=3
  BusInP : BusCreator  Inputs=2
  BusState : BusCreator  Inputs=2
  LLMon : Outport
  wires:
  [InPMon] -> Bus/1
  [StateMon] -> Bus/2
  LKAMon/1 -> Bus/3
  Bus/1 -> LLMon/1  "LLMon"
  [LFTTTLC_Mon] -> BusInP/1  "LFTTTLC_Mon"
  [RGTTTLC_Mon] -> BusInP/2  "RGTTTLC_Mon"
  [LDW_State_Mon] -> BusState/1  "LDW_State_Mon"
  [LKA_State_Mon] -> BusState/2  "LKA_State_Mon"
  BusInP/1 -> [InPMon]  "InPMon"
  BusState/1 -> [StateMon]  "StateMon"

== system LKAS_DFL_20210630/LKAS/LL/LLOut/Angle2Trq ==
  LKA_Torque_Req : Inport
  Target_Angle : Inport  Port=2
  Stearing_Angle : Inport  Port=3
  Constant : Constant  Value=5  OutDataTypeStr=single
  Constant1 : Constant  Value=-5  OutDataTypeStr=single
  Constant3 : Constant  Value=5  OutDataTypeStr=single
  Constant4 : Constant  Value=-5  OutDataTypeStr=single
  Rate Limiter Dynamic : Subsystem
  Saturation Dynamic : Subsystem
  Subsystem : Subsystem
  torque : Outport  OutputWhenDisabled=reset  InitialOutput=0
  wires:
  Saturation Dynamic/1(y) -> torque/1  "Saturation_trq"
  Constant4/1 -> Saturation Dynamic/3(lo)
  Constant3/1 -> Saturation Dynamic/1(up)
  Rate Limiter Dynamic/1(Y) -> Saturation Dynamic/2(u)  "RL_trq"
  Constant1/1 -> Rate Limiter Dynamic/3(lo)
  Constant/1 -> Rate Limiter Dynamic/1(up)
  Target_Angle/1 -> Subsystem/1(Target_Angle)  "Target_Angle"
  Stearing_Angle/1 -> Subsystem/2(Stearing_Angle)  "Stearing_Angle"
  Subsystem/1(in_trq) -> Rate Limiter Dynamic/2(u)  "in_trq"
  LKA_Torque_Req/1 -> Subsystem/Enable  "LKA_Torque_Req"

== system LKAS_DFL_20210630/LKAS/LLClb/LLSMConClb/ICv to v10 ==
  In1 : Inport
  Add : Sum  Inputs=+-
  Constant : Constant  Value=2.5  OutDataTypeStr=single
  Gain : Gain  Gain=1/1.02
  Out1 : Outport
  wires:
  In1/1 -> Add/1
  Add/1 -> Gain/1
  Constant/1 -> Add/2
  Gain/1 -> Out1/1

== system LKAS_DFL_20210630/LKAS/LLClb/LLSMConClb/ICv to v11 ==
  In1 : Inport
  Add : Sum  Inputs=+-
  Constant : Constant  Value=2.5  OutDataTypeStr=single
  Gain : Gain  Gain=1/1.02
  Out1 : Outport
  wires:
  Gain/1 -> Out1/1
  Constant/1 -> Add/2
  Add/1 -> Gain/1
  In1/1 -> Add/1

== system LKAS_DFL_20210630/LKAS/LLClb/LLSMConClb/ICv to v6 ==
  In1 : Inport
  Add : Sum  Inputs=+-
  Constant : Constant  Value=2.5  OutDataTypeStr=single
  Gain : Gain  Gain=1/1.02
  Out1 : Outport
  wires:
  In1/1 -> Add/1
  Add/1 -> Gain/1
  Constant/1 -> Add/2
  Gain/1 -> Out1/1

== system LKAS_DFL_20210630/LKAS/LLClb/LLSMConClb/ICv to v7 ==
  In1 : Inport
  Add : Sum  Inputs=+-
  Constant : Constant  Value=2.5  OutDataTypeStr=single
  Gain : Gain  Gain=1/1.02
  Out1 : Outport
  wires:
  Gain/1 -> Out1/1
  Constant/1 -> Add/2
  Add/1 -> Gain/1
  In1/1 -> Add/1

== system LKAS_DFL_20210630/LKAS/LLClb/LLSMConClb/ICv to v8 ==
  In1 : Inport
  Add : Sum  Inputs=+-
  Constant : Constant  Value=2.5  OutDataTypeStr=single
  Gain : Gain  Gain=1/1.02
  Out1 : Outport
  wires:
  In1/1 -> Add/1
  Add/1 -> Gain/1
  Constant/1 -> Add/2
  Gain/1 -> Out1/1

== system LKAS_DFL_20210630/LKAS/LLClb/LLSMConClb/ICv to v9 ==
  In1 : Inport
  Add : Sum  Inputs=+-
  Constant : Constant  Value=2.5  OutDataTypeStr=single
  Gain : Gain  Gain=1/1.02
  Out1 : Outport
  wires:
  Gain/1 -> Out1/1
  Constant/1 -> Add/2
  Add/1 -> Gain/1
  In1/1 -> Add/1

== system LKAS_DFL_20210630/LKAS/LL/HMI/Subsystem/Count 10s ==
  Enable : EnablePort  StatesWhenEnabling=reset
      settings: AttributesFormatString=states = %<StatesWhenEnabling>
  Add : Sum
  Compare To Constant27 : simulink/Logic and Bit Operations/Compare To Constant  relop=>=  const=1000  OutDataTypeStr=boolean
  Constant : Constant  OutDataTypeStr=uint16
  Memory : Memory  InheritSampleTime=on
  Saturation : Saturate  UpperLimit=2100  LowerLimit=0
      settings: AttributesFormatString="Min = %<LowerLimit>  Max = %<UpperLimit>"
  Out : Outport  OutputWhenDisabled=reset  InitialOutput=0
      settings: AttributesFormatString=%<OutputWhenDisabled> = %<InitialOutput>
  wires:
  Compare To Constant27/1 -> Out/1
  Constant/1 -> Add/1
  Add/1 -> Saturation/1
  Saturation/1 -> Compare To Constant27/1, Memory/1
  Memory/1 -> Add/2

== system LKAS_DFL_20210630/LKAS/LL/HMI/Subsystem/Count 15s ==
  Enable : EnablePort  StatesWhenEnabling=reset
      settings: AttributesFormatString=states = %<StatesWhenEnabling>
  Add : Sum
  Compare To Constant27 : simulink/Logic and Bit Operations/Compare To Constant  relop=>=  const=1500  OutDataTypeStr=boolean
  Constant : Constant  OutDataTypeStr=uint16
  Memory : Memory  InheritSampleTime=on
  Saturation : Saturate  UpperLimit=2100  LowerLimit=0
      settings: AttributesFormatString="Min = %<LowerLimit>  Max = %<UpperLimit>"
  Out : Outport  OutputWhenDisabled=reset  InitialOutput=0
      settings: AttributesFormatString=%<OutputWhenDisabled> = %<InitialOutput>
  wires:
  Memory/1 -> Add/2
  Saturation/1 -> Memory/1, Compare To Constant27/1
  Add/1 -> Saturation/1
  Constant/1 -> Add/1
  Compare To Constant27/1 -> Out/1

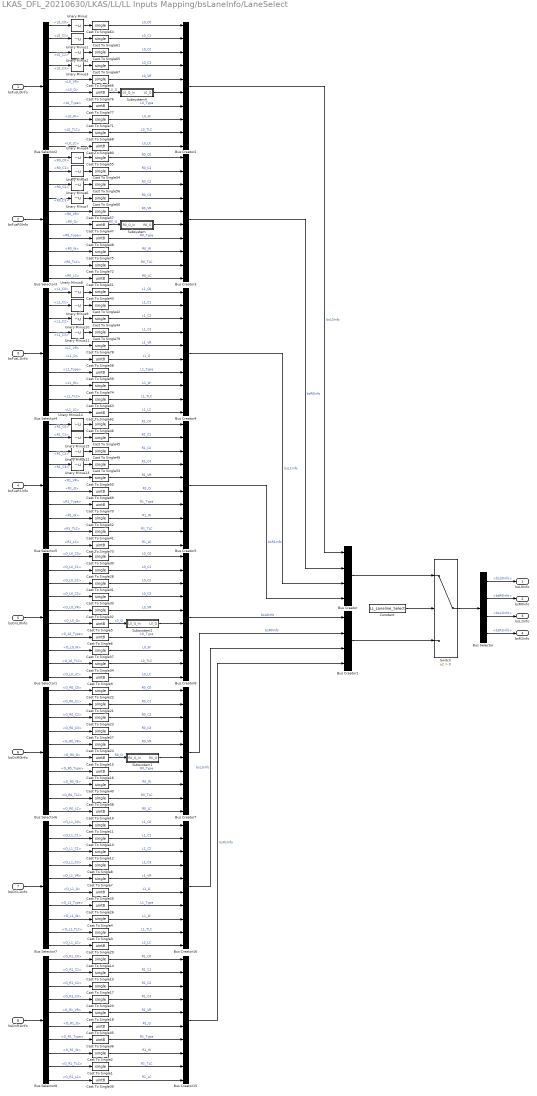
== system LKAS_DFL_20210630/LKAS/LL/LL Inputs Mapping/bsLaneInfo/LaneSelect ==
  bsFusL0Info : Inport
  bsFusR0Info : Inport  Port=2
  bsFusL1Info : Inport  Port=3
  bsFusR1Info : Inport  Port=4
  bsOriL0Info : Inport  Port=5
  bsOriR0Info : Inport  Port=6
  bsOriL1Info : Inport  Port=7
  bsOriR1Info : Inport  Port=8
  Bus Creator : BusCreator  Inputs=4
  Bus Creator1 : BusCreator  Inputs=4
  Bus Creator{2..5,7..8,15..16} (8 alike) : BusCreator  Inputs=10
  Bus Selector : BusSelector  OutputSignals=bsL0Info,bsR0Info,bsL1Info,bsR1Info
  Bus Selector1 : BusSelector  OutputSignals=O_L0_C0,O_L0_C1,O_L0_C2,O_L0_C3,O_L0_VR,O_L0_Q,O_L0_Type,O_L0_W,O_L0_TLC,O_L0_LC
  Bus Selector2 : BusSelector  OutputSignals=L0_C0,L0_C1,L0_C2,L0_C3,L0_VR,L0_Q,L0_Type,L0_W,L0_TLC,L0_LC
  Bus Selector3 : BusSelector  OutputSignals=R0_C0,R0_C1,R0_C2,R0_C3,R0_VR,R0_Q,R0_Type,R0_W,R0_TLC,R0_LC
  Bus Selector4 : BusSelector  OutputSignals=L1_C0,L1_C1,L1_C2,L1_C3,L1_VR,L1_Q,L1_Type,L1_W,L1_TLC,L1_LC
  Bus Selector5 : BusSelector  OutputSignals=R1_C0,R1_C1,R1_C2,R1_C3,R1_VR,R1_Q,R1_Type,R1_W,R1_TLC,R1_LC
  Bus Selector6 : BusSelector  OutputSignals=O_R0_C0,O_R0_C1,O_R0_C2,O_R0_C3,O_R0_VR,O_R0_Q,O_R0_Type,O_R0_W,O_R0_TLC,O_R0_LC
  Bus Selector7 : BusSelector  OutputSignals=O_L1_C0,O_L1_C1,O_L1_C2,O_L1_C3,O_L1_VR,O_L1_Q,O_L1_Type,O_L1_W,O_L1_TLC,O_L1_LC
  Bus Selector8 : BusSelector  OutputSignals=O_R1_C0,O_R1_C1,O_R1_C2,O_R1_C3,O_R1_VR,O_R1_Q,O_R1_Type,O_R1_W,O_R1_TLC,O_R1_LC
  Cast To Single{1..4,7..8,10..14,17..18,20..24,27..28,30..34,37..38,40..46,49..50,52..57,60..61,63..68,71..72,74..75,78..79} (56 alike) : DataTypeConversion  OutDataTypeStr=single
  Cast To Single{5..6,9,15..16,19,25..26,29,35..36,39,47..48,51,58..59,62,69..70,73,76..77,80} (24 alike) : DataTypeConversion  OutDataTypeStr=uint8
  Constant : Constant  Value=LL_Laneline_Select  OutDataTypeStr=single
  Subsystem : Subsystem
  Subsystem1 : Subsystem
  Subsystem2 : Subsystem
  Subsystem4 : Subsystem
  Switch : Switch  Criteria=u2 > Threshold
  Unary Minus{,1..15} (16 alike) : UnaryMinus
  bsL0Info : Outport
  bsR0Info : Outport  Port=2
  bsL1Info : Outport  Port=3
  bsR1Info : Outport  Port=4
  wires:
  Subsystem1/1(R0_Q) -> Bus Creator7/6
  Subsystem2/1(L0_Q) -> Bus Creator8/6
  Bus Selector/4 -> bsR1Info/1  "<bsR1Info>"
  Bus Selector/3 -> bsL1Info/1  "<bsL1Info>"
  Bus Selector/2 -> bsR0Info/1  "<bsR0Info>"
  Bus Selector/1 -> bsL0Info/1  "<bsL0Info>"
  Bus Selector4/3 -> Unary Minus10/1  "<L1_C2>"
  Bus Selector4/8 -> Cast To Single74/1  "<L1_W>"
  Bus Selector5/3 -> Unary Minus12/1  "<R1_C2>"
  Bus Selector5/2 -> Unary Minus15/1  "<R1_C1>"
  Bus Selector5/8 -> Cast To Single52/1  "<R1_W>"
  Bus Creator5/1 -> Bus Creator/4  "bsR1Info"
  Bus Selector5/4 -> Unary Minus13/1  "<R1_C3>"
  Bus Selector5/9 -> Cast To Single41/1  "<R1_TLC>"
  Bus Selector3/6 -> Cast To Single47/1  "<R0_Q>"
  Subsystem/1(R0_Q) -> Bus Creator3/6
  Bus Selector2/7 -> Cast To Single77/1  "<L0_Type>"
  Bus Selector4/9 -> Cast To Single63/1  "<L1_TLC>"
  Bus Selector4/6 -> Cast To Single58/1  "<L1_Q>"
  Bus Selector4/4 -> Unary Minus11/1  "<L1_C3>"
  Bus Selector2/2 -> Unary Minus1/1  "<L0_C1>"
  Bus Selector3/1 -> Unary Minus4/1  "<R0_C0>"
  Bus Selector3/2 -> Unary Minus5/1  "<R0_C1>"
  Bus Selector2/8 -> Cast To Single71/1  "<L0_W>"
  Bus Selector3/4 -> Unary Minus7/1  "<R0_C3>"
  Bus Selector4/10 -> Cast To Single62/1  "<L1_LC>"
  Bus Selector2/1 -> Unary Minus/1  "<L0_C0>"
  Bus Selector2/5 -> Cast To Single66/1  "<L0_VR>"
  Bus Selector5/5 -> Cast To Single50/1  "<R1_VR>"
  Bus Selector5/6 -> Cast To Single69/1  "<R1_Q>"
  Bus Selector2/9 -> Cast To Single68/1  "<L0_TLC>"
  Bus Selector5/7 -> Cast To Single70/1  "<R1_Type>"
  Bus Selector2/10 -> Cast To Single80/1  "<L0_LC>"
  Bus Selector3/3 -> Unary Minus6/1  "<R0_C2>"
  Bus Selector3/9 -> Cast To Single72/1  "<R0_TLC>"
  Bus Selector3/7 -> Cast To Single48/1  "<R0_Type>"
  Bus Selector3/8 -> Cast To Single75/1  "<R0_W>"
  Bus Selector5/1 -> Unary Minus14/1  "<R1_C0>"
  Bus Selector2/3 -> Unary Minus2/1  "<L0_C2>"
  Bus Selector5/10 -> Cast To Single73/1  "<R1_LC>"
  Bus Selector3/10 -> Cast To Single51/1  "<R0_LC>"
  bsFusL0Info/1 -> Bus Selector2/1
  Bus Selector4/7 -> Cast To Single59/1  "<L1_Type>"
  bsFusR0Info/1 -> Bus Selector3/1
  bsFusL1Info/1 -> Bus Selector4/1
  bsFusR1Info/1 -> Bus Selector5/1
  Bus Selector2/6 -> Cast To Single76/1  "<L0_Q>"
  Bus Selector2/4 -> Unary Minus3/1  "<L0_C3>"
  Bus Selector4/1 -> Unary Minus8/1  "<L1_C0>"
  Subsystem4/1(L0_Q) -> Bus Creator2/6
  Bus Selector3/5 -> Cast To Single57/1  "<R0_VR>"
  Bus Selector4/2 -> Unary Minus9/1  "<L1_C1>"
  Bus Selector4/5 -> Cast To Single78/1  "<L1_VR>"
  Switch/1 -> Bus Selector/1
  Constant/1 -> Switch/2
  Bus Creator1/1 -> Switch/3
  Bus Creator/1 -> Switch/1
  Bus Creator4/1 -> Bus Creator/3  "bsL1Info"
  Bus Creator3/1 -> Bus Creator/2  "bsR0Info"
  Bus Creator2/1 -> Bus Creator/1  "bsL0Info"
  Bus Selector8/10 -> Cast To Single39/1  "<O_R1_LC>"
  Bus Selector8/9 -> Cast To Single1/1  "<O_R1_TLC>"
  Bus Selector8/8 -> Cast To Single2/1  "<O_R1_W>"
  Bus Selector8/7 -> Cast To Single36/1  "<O_R1_Type>"
  Bus Selector8/6 -> Cast To Single35/1  "<O_R1_Q>"
  Bus Selector8/5 -> Cast To Single18/1  "<O_R1_VR>"
  Bus Selector8/4 -> Cast To Single20/1  "<O_R1_C3>"
  Bus Selector8/3 -> Cast To Single17/1  "<O_R1_C2>"
  Bus Selector8/2 -> Cast To Single13/1  "<O_R1_C1>"
  Bus Selector8/1 -> Cast To Single14/1  "<O_R1_C0>"
  bsOriR1Info/1 -> Bus Selector8/1
  Bus Selector7/10 -> Cast To Single29/1  "<O_L1_LC>"
  Bus Selector7/9 -> Cast To Single3/1  "<O_L1_TLC>"
  Bus Selector7/8 -> Cast To Single4/1  "<O_L1_W>"
  Bus Selector7/7 -> Cast To Single26/1  "<O_L1_Type>"
  Bus Selector7/6 -> Cast To Single25/1  "<O_L1_Q>"
  Bus Selector7/5 -> Cast To Single7/1  "<O_L1_VR>"
  Bus Selector7/4 -> Cast To Single8/1  "<O_L1_C3>"
  Bus Selector7/3 -> Cast To Single12/1  "<O_L1_C2>"
  Bus Selector7/2 -> Cast To Single10/1  "<O_L1_C1>"
  Bus Selector7/1 -> Cast To Single11/1  "<O_L1_C0>"
  bsOriL1Info/1 -> Bus Selector7/1
  Bus Selector6/10 -> Cast To Single19/1  "<O_R0_LC>"
  Bus Selector6/9 -> Cast To Single38/1  "<O_R0_TLC>"
  Bus Selector6/8 -> Cast To Single40/1  "<O_R0_W>"
  Bus Selector6/7 -> Cast To Single16/1  "<O_R0_Type>"
  Bus Selector6/6 -> Cast To Single15/1  "<O_R0_Q>"
  Bus Selector6/5 -> Cast To Single24/1  "<O_R0_VR>"
  Bus Selector6/4 -> Cast To Single27/1  "<O_R0_C3>"
  Bus Selector6/3 -> Cast To Single23/1  "<O_R0_C2>"
  Bus Selector6/2 -> Cast To Single21/1  "<O_R0_C1>"
  Bus Selector6/1 -> Cast To Single22/1  "<O_R0_C0>"
  bsOriR0Info/1 -> Bus Selector6/1
  Bus Selector1/10 -> Cast To Single9/1  "<O_L0_LC>"
  Bus Selector1/9 -> Cast To Single34/1  "<O_L0_TLC>"
  Bus Selector1/8 -> Cast To Single37/1  "<O_L0_W>"
  Bus Selector1/7 -> Cast To Single6/1  "<O_L0_Type>"
  Bus Selector1/6 -> Cast To Single5/1  "<O_L0_Q>"
  Bus Selector1/5 -> Cast To Single32/1  "<O_L0_VR>"
  Bus Selector1/4 -> Cast To Single33/1  "<O_L0_C3>"
  Bus Selector1/3 -> Cast To Single31/1  "<O_L0_C2>"
  Bus Selector1/2 -> Cast To Single28/1  "<O_L0_C1>"
  Bus Selector1/1 -> Cast To Single30/1  "<O_L0_C0>"
  bsOriL0Info/1 -> Bus Selector1/1
  Cast To Single2/1 -> Bus Creator15/8  "R1_W"
  Cast To Single27/1 -> Bus Creator7/4  "R0_C3"
  Cast To Single10/1 -> Bus Creator16/2  "L1_C1"
  Cast To Single32/1 -> Bus Creator8/5  "L0_VR"
  Cast To Single37/1 -> Bus Creator8/8  "L0_W"
  Cast To Single40/1 -> Bus Creator7/8  "R0_W"
  Bus Creator8/1 -> Bus Creator1/1  "bsL0Info"
  Cast To Single22/1 -> Bus Creator7/1  "R0_C0"
  Cast To Single25/1 -> Bus Creator16/6  "L1_Q"
  Cast To Single17/1 -> Bus Creator15/3  "R1_C2"
  Cast To Single36/1 -> Bus Creator15/7  "R1_Type"
  Cast To Single9/1 -> Bus Creator8/10  "L0_LC"
  Cast To Single31/1 -> Bus Creator8/3  "L0_C2"
  Cast To Single30/1 -> Bus Creator8/1  "L0_C0"
  Cast To Single33/1 -> Bus Creator8/4  "L0_C3"
  Cast To Single5/1 -> Subsystem2/1(L0_Q_In)  "L0_Q"
  Cast To Single6/1 -> Bus Creator8/7  "L0_Type"
  Cast To Single16/1 -> Bus Creator7/7  "R0_Type"
  Cast To Single35/1 -> Bus Creator15/6  "R1_Q"
  Cast To Single28/1 -> Bus Creator8/2  "L0_C1"
  Cast To Single1/1 -> Bus Creator15/9  "R1_TLC"
  Cast To Single21/1 -> Bus Creator7/2  "R0_C1"
  Cast To Single23/1 -> Bus Creator7/3  "R0_C2"
  Bus Creator16/1 -> Bus Creator1/3  "bsL1Info"
  Cast To Single13/1 -> Bus Creator15/2  "R1_C1"
  Cast To Single14/1 -> Bus Creator15/1  "R1_C0"
  Cast To Single26/1 -> Bus Creator16/7  "L1_Type"
  Cast To Single20/1 -> Bus Creator15/4  "R1_C3"
  Cast To Single24/1 -> Bus Creator7/5  "R0_VR"
  Cast To Single7/1 -> Bus Creator16/5  "L1_VR"
  Cast To Single15/1 -> Subsystem1/1(R0_Q_In)  "R0_Q"
  Cast To Single11/1 -> Bus Creator16/1  "L1_C0"
  Cast To Single38/1 -> Bus Creator7/9  "R0_TLC"
  Cast To Single4/1 -> Bus Creator16/8  "L1_W"
  Cast To Single12/1 -> Bus Creator16/3  "L1_C2"
  Cast To Single19/1 -> Bus Creator7/10  "R0_LC"
  Cast To Single39/1 -> Bus Creator15/10  "R1_LC"
  Cast To Single18/1 -> Bus Creator15/5  "R1_VR"
  Cast To Single3/1 -> Bus Creator16/9  "L1_TLC"
  Cast To Single29/1 -> Bus Creator16/10  "L1_LC"
  Cast To Single8/1 -> Bus Creator16/4  "L1_C3"
  Bus Creator15/1 -> Bus Creator1/4  "bsR1Info"
  Cast To Single34/1 -> Bus Creator8/9  "L0_TLC"
  Bus Creator7/1 -> Bus Creator1/2  "bsR0Info"
  Cast To Single61/1 -> Bus Creator2/2  "L0_C1"
  Cast To Single66/1 -> Bus Creator2/5  "L0_VR"
  Cast To Single67/1 -> Bus Creator2/4  "L0_C3"
  Cast To Single65/1 -> Bus Creator2/3  "L0_C2"
  Cast To Single64/1 -> Bus Creator2/1  "L0_C0"
  Cast To Single76/1 -> Subsystem4/1(L0_Q_In)  "L0_Q"
  Cast To Single68/1 -> Bus Creator2/9  "L0_TLC"
  Cast To Single77/1 -> Bus Creator2/7  "L0_Type"
  Cast To Single80/1 -> Bus Creator2/10  "L0_LC"
  Cast To Single56/1 -> Bus Creator3/3  "R0_C2"
  Cast To Single54/1 -> Bus Creator3/2  "R0_C1"
  Cast To Single55/1 -> Bus Creator3/1  "R0_C0"
  Cast To Single47/1 -> Subsystem/1(R0_Q_In)  "R0_Q"
  Cast To Single48/1 -> Bus Creator3/7  "R0_Type"
  Cast To Single51/1 -> Bus Creator3/10  "R0_LC"
  Cast To Single57/1 -> Bus Creator3/5  "R0_VR"
  Cast To Single60/1 -> Bus Creator3/4  "R0_C3"
  Cast To Single72/1 -> Bus Creator3/9  "R0_TLC"
  Cast To Single75/1 -> Bus Creator3/8  "R0_W"
  Cast To Single44/1 -> Bus Creator4/3  "L1_C2"
  Cast To Single58/1 -> Bus Creator4/6  "L1_Q"
  Cast To Single59/1 -> Bus Creator4/7  "L1_Type"
  Cast To Single43/1 -> Bus Creator4/1  "L1_C0"
  Cast To Single42/1 -> Bus Creator4/2  "L1_C1"
  Cast To Single78/1 -> Bus Creator4/5  "L1_VR"
  Cast To Single79/1 -> Bus Creator4/4  "L1_C3"
  Cast To Single62/1 -> Bus Creator4/10  "L1_LC"
  Cast To Single63/1 -> Bus Creator4/9  "L1_TLC"
  Cast To Single74/1 -> Bus Creator4/8  "L1_W"
  Cast To Single45/1 -> Bus Creator5/2  "R1_C1"
  Cast To Single46/1 -> Bus Creator5/1  "R1_C0"
  Cast To Single49/1 -> Bus Creator5/3  "R1_C2"
  Cast To Single50/1 -> Bus Creator5/5  "R1_VR"
  Cast To Single52/1 -> Bus Creator5/8  "R1_W"
  Cast To Single53/1 -> Bus Creator5/4  "R1_C3"
  Cast To Single41/1 -> Bus Creator5/9  "R1_TLC"
  Cast To Single69/1 -> Bus Creator5/6  "R1_Q"
  Cast To Single70/1 -> Bus Creator5/7  "R1_Type"
  Cast To Single73/1 -> Bus Creator5/10  "R1_LC"
  Cast To Single71/1 -> Bus Creator2/8  "L0_W"
  Unary Minus/1 -> Cast To Single64/1
  Unary Minus1/1 -> Cast To Single61/1
  Unary Minus2/1 -> Cast To Single65/1
  Unary Minus3/1 -> Cast To Single67/1
  Unary Minus7/1 -> Cast To Single60/1
  Unary Minus6/1 -> Cast To Single56/1
  Unary Minus4/1 -> Cast To Single55/1
  Unary Minus5/1 -> Cast To Single54/1
  Unary Minus8/1 -> Cast To Single43/1
  Unary Minus9/1 -> Cast To Single42/1
  Unary Minus11/1 -> Cast To Single79/1
  Unary Minus10/1 -> Cast To Single44/1
  Unary Minus12/1 -> Cast To Single49/1
  Unary Minus13/1 -> Cast To Single53/1
  Unary Minus14/1 -> Cast To Single46/1
  Unary Minus15/1 -> Cast To Single45/1
